simulink model "NonLinearDroopControlExample"  (R2021a)
settings: Solver=VariableStepAuto  StartTime=0.0  StopTime=20  RelTol=1e-3
libraries: simulink x1
settings Model: Creator=Sajid Ali  LastModifiedBy=Sajid Ali

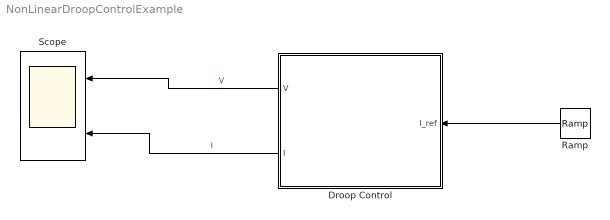
== system NonLinearDroopControlExample ==
  Droop Control : Subsystem  mask{Irated=10, Vnom=120, Vrated=100, alpha=3}
      mask prompts: Irated "Maximum Current (A)"; Vnom "Maximum Voltage (V)"; Vrated "Minimum Voltage (V)"; alpha "Arc Coefficient(alpha)"
      mask init:
      | m=(Vnom-Vrated)/((2*Irated)^alpha);
      mask DialogControl DescGroupVar Prompt: Description about the block
      mask DialogControl DescTextVar Prompt: This block implements a linear droop control with saturation limit on input current Author:sajidali
  Ramp : simulink/Sources/Ramp  slope=1  start=0  InitialOutput=-10
  Scope : Scope  NumInputPorts=2
  wires:
  Ramp/1 -> Droop Control/1(I_ref)
  Droop Control/1(V) -> Scope/1  "V"
  Droop Control/2(I) -> Scope/2  "I"

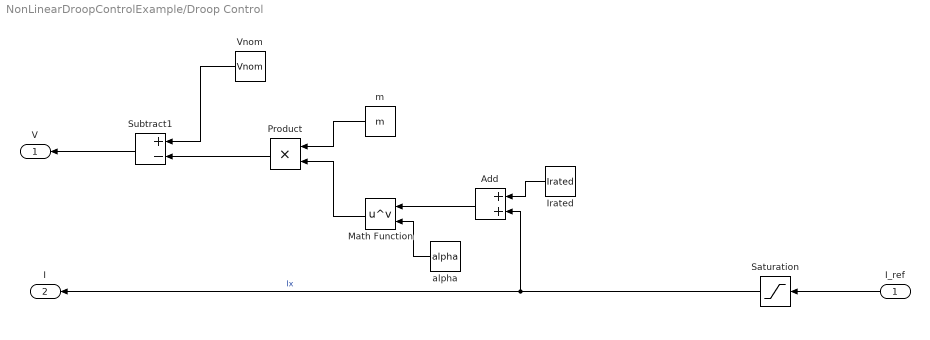
== system NonLinearDroopControlExample/Droop Control ==
  I_ref : Inport
  Add : Sum
  Irated : Constant  Value=Irated
  Math Function : Math  Operator=pow  SaturateOnIntegerOverflow=on
  Product : Product
  Saturation : Saturate  UpperLimit=Irated  LowerLimit=-Irated
  Subtract1 : Sum  Inputs=+-
  Vnom : Constant  Value=Vnom
  alpha : Constant  Value=alpha
  m : Constant  Value=m
  V : Outport
  I : Outport  Port=2
  wires:
  Product/1 -> Subtract1/2
  Vnom/1 -> Subtract1/1
  m/1 -> Product/1
  Saturation/1 -> Add/2, I/1  "Ix"
  Subtract1/1 -> V/1
  I_ref/1 -> Saturation/1
  Irated/1 -> Add/1
  Add/1 -> Math Function/1
  alpha/1 -> Math Function/2
  Math Function/1 -> Product/2
